simulink model "mehrw1"  (Simulink 4.00)
settings: Solver=ode45  SolverMode=SingleTasking  StartTime=0.0  StopTime=30  FixedStep=0.1  MaxStep=0.1  RelTol=1e-3  AbsTol=1e-6
values from neighbouring files (symbols this model uses):
  rT = 0.1    [mehrw_1.m]    (also in mehrw_2.m; mehrw_3.m; mehrw_4.m; mehrw_5.m)
settings Model: LastModifiedBy=Administrator  Refine=3  SaveTime=off  SaveOutput=off  LimitDataPoints=off  BlockReductionOpt=off

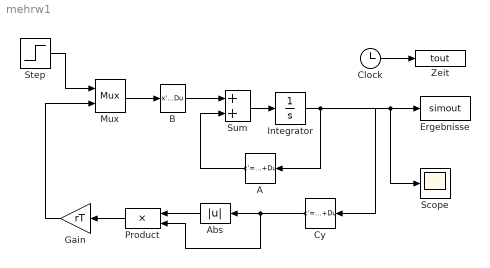
== system mehrw1 ==
  A : StateSpace  Orientation=left  A=[]  B=[]  C=[]  D=K  X0=0  Realization=auto  AbsoluteTolerance=auto  mask(Matrix Gain){@1=A}
      mask prompts: @1 "Gain matrix:"
      mask help: Matrix Gain.
      mask init:
      | K = @1;
      mask Help: Multiplies input vector by entered matrix to produce output vector (y=Au).
      mask Display: disp('K')
  Abs : Abs  Orientation=left  SaturateOnIntegerOverflow=on
  B : StateSpace  A=[]  B=[]  C=[]  D=K  X0=0  Realization=auto  AbsoluteTolerance=auto  mask(Matrix Gain){@1=B}
      mask prompts: @1 "Gain matrix:"
      mask help: Matrix Gain.
      mask init:
      | K = @1;
      mask Help: Multiplies input vector by entered matrix to produce output vector (y=Au).
      mask Display: disp('K')
  Clock : Clock
      settings: DisplayTime=off  Decimation=10
  Cy : StateSpace  Orientation=left  A=[]  B=[]  C=[]  D=K  X0=0  Realization=auto  AbsoluteTolerance=auto  mask(Matrix Gain){@1=Cy}
      mask prompts: @1 "Gain matrix:"
      mask help: Matrix Gain.
      mask init:
      | K = @1;
      mask Help: Multiplies input vector by entered matrix to produce output vector (y=Au).
      mask Display: disp('K')
  Ergebnisse : ToWorkspace  VariableName=simout  SampleTime=0  SaveFormat=Array
      settings: MaxDataPoints=1000
  Gain : Gain  Orientation=left  Gain=rT  Multiplication=Element-wise(K.*u)  SaturateOnIntegerOverflow=on
  Integrator : Integrator  ExternalReset=none  InitialConditionSource=internal  InitialCondition=[0 0 0 0 0 1 0 0 0 0]  LimitOutput=off  UpperSaturationLimit=inf  LowerSaturationLimit=-inf  ShowSaturationPort=off  ShowStatePort=off  AbsoluteTolerance=auto
  Mux : Mux  Inputs=2
      settings: DisplayOption=none
  Product : Product  Orientation=left  Inputs=2  Multiplication=Element-wise(.*)  SaturateOnIntegerOverflow=on
  Scope : Scope
      settings: TickLabels=on  TimeRange=30  YMin=-41.6038  YMax=41.6038  SaveToWorkspace=off  SaveName=ScopeData  DataFormat=Array  LimitDataPoints=on  MaxDataPoints=5000
  Step : Step  Time=0  Before=0  After=1  SampleTime=0
  Sum : Sum  Inputs=++  SaturateOnIntegerOverflow=on
  Zeit : ToWorkspace  VariableName=tout  SampleTime=0  SaveFormat=Array
      settings: MaxDataPoints=1000
  wires:
  Cy/1 -> Product/2, Abs/1
  Product/1 -> Gain/1
  Gain/1 -> Mux/2
  Abs/1 -> Product/1
  Integrator/1 -> Scope/1, Ergebnisse/1, Cy/1, A/1
  A/1 -> Sum/2
  Step/1 -> Mux/1
  B/1 -> Sum/1
  Sum/1 -> Integrator/1
  Mux/1 -> B/1
  Clock/1 -> Zeit/1
